simulink model "sim_5_twolink_force_control"  (R2021a)
settings: Solver=VariableStepAuto  StartTime=0.0  StopTime=15  MaxStep=1e-2
values from neighbouring files (symbols this model uses):
  b1 = 0.01    [sim_params.m]    (also in sim_params_force.m)
  b2 = 0.01    [sim_params.m]    (also in sim_params_force.m)
  D = [zeros(n); eye(n)]    [control_comparison_script.m]    (also in gen_twolink_ss.m = reshape([0.0,0.0,0.0,0.0,0.0,0.0,0.0,0.0],[4,2]))
  g = 9.80665    [sim_params.m]    (also in sim_params_force.m)
  L1x = 0.3    [sim_params.m]    (also in sim_params_force.m)
  L1y = 0.050    (= 0.05)    [sim_params.m]    (also in sim_params_force.m)
  L1z = 0.05    [sim_params.m]    (also in sim_params_force.m)
  L2x = 0.15    [sim_params.m]    (also in sim_params_force.m = 0.3)
  L2y = 0.05    [sim_params.m]    (also in sim_params_force.m)
  L2z = 0.05    [sim_params.m]    (also in sim_params_force.m)
  m1 = m1*1.25    [control_comparison_script.m]    (also in sim_params.m = 2.775; sim_params_force.m = 2.775)
  m2 = m2*1.25    [control_comparison_script.m]    (also in sim_params.m = 1.3875; sim_params_force.m = 2.775)
  max_joint_torque1 = 20    [sim_params.m]    (also in sim_params_force.m)
  max_joint_torque2 = 10    [sim_params.m]    (also in sim_params_force.m = 20)
undefined symbols (not defined in the file or in its folder): Da, KD, KD_a, Kd_p, Kd_p2, Kdt, KF, Kf_v, Kf_v2, KI, Ki_f, Ki_f2, Ki_p, Ki_p2, KP, KP_a, Kp_f, Kp_f2, Kp_p, Kp_p2, Levenberg, Ma, Marquardt, R_env, sigbuilder_block, W_env, X, Xenv, Y, Z
libraries: sm_lib x72, nesl_utility x58, pid_lib x14, simulink x3, robotmaniplib x2, robotcorelib x1
(part 1 of 6)
settings Model: Creator=Petronas-Tareq  LastModifiedBy=Petronas-Tareq
settings ExplorerConfigSet: InternalSimMechanicsExplorerSettings="<ExplorerConfiguration><canonicalview>default</canonicalview><AnimationSetting><BasePlaybackSpeed>1.0</BasePlaybackSpeed><PlaybackSpeedFactor>1.0</PlaybackSpeedFactor></AnimationSetting><TilePanel><TileInfo><Tiles Columns=\"2\" Count=\"4\" Rows=\"2\"><Column Weight=\"0.4998\"/><Column Weight=\"0.5002\"/><Row Weight=\"0.5\"/><Row Weight=\"0.5\"/><Tile Height=\"1\" Width=\"1\" X=\"0\" Y=\"0\"/><Tile Height=\"1\" Width=\"1\" X=\"0\" Y=\"1\"/><Tile Height=\"1\" Width=\"1\" X=\"1\" Y=\"0\"/><Tile Height=\"1\" Width=\"1\" X=\"1\" Y=\"1\"/></Tiles></TileInfo><SceneInfo><SceneViewer><BGColor><R>0.60000002384185791</R><G>0.60000002384185791</G><B>0.60000002384185791</B></BGColor><Camera><DoPerspective>off</DoPerspective><Position><X>0.22866161329300444</X><Y>-0.999999955971509147</Y><Z>-4.12820655437684536e-09</Z></Position><Center><X>0.22866161329300444</X><Y>4.40284908531651742e-08</Y><Z>-4.12820655437684536e-09</Z></Center><Up><X>0</X><Y>-0</Y><Z>1</Z></Up><ViewLimDist>1</ViewLimDist><YLim>0.367330397528709274</YLim><XLim>0.552253577106518345</XLim></Camera></SceneViewer><SceneViewer><BGColor><R>0.60000002384185791</R><G>0.60000002384185791</G><B>0.60000002384185791</B></BGColor><Camera><DoPerspective>off</DoPerspective><Position><X>0.204072367525804987</X><Y>-2.34335064047906805</Y><Z>0.167988192192854713</Z></Position><Center><X>0.219660802383778442</X><Y>-1.34642671678176962</Y><Z>0.0911787457755401237</Z></Center><Up><X>-0.0262288638413234881</X><Y>0.0772000539040926803</Y><Z>0.996670556592697987</Z></Up><ViewLimDist>1</ViewLimDist><YLim>0.734660795057418547</YLim><XLim>1.10450715421303669</XLim></Camera></SceneViewer><SceneViewer><BGColor><R>0.60000002384185791</R><G>0.60000002384185791</G><B>0.60000002384185791</B></BGColor><Camera><DoPerspective>off</DoPerspective><Position><X>-0.24899486320315789</X><Y>-0.765272772333560392</Y><Z>0.697835060620221048</Z></Position><Center><X>0.26973731486207464</X><Y>-0.211131790133127217</Y><Z>0.0468014982858467876</Z></Center><Up><X>0.244353234025975474</X><Y>0.633635300715601257</Y><Z>0.734028475406845016</Z></Up><ViewLimDist>1</ViewLimDist><YLim>0.614833162544433431</YLim><XLim>0.925057201179866673</XLim></Camera></SceneViewer><SceneViewer><BGColor><R>0.60000002384185791</R><G>0.60000002384185791</G><B>0.60000002384185791</B></BGColor><Camera><DoPerspective>off</DoPerspective><Position><X>0.236408339938699752</X><Y>-3.48082895840207129e-09</Y><Z>0.999999999307370047</Z></Position><Center><X>0.236408339938699752</X><Y>-3.48082895840207129e-09</Y><Z>-6.9262995339158806e-10</Z></Center><Up><X>0</X><Y>1</Y><Z>-0</Z></Up><ViewLimDist>1</ViewLimDist><YLim>0.734647572682027739</YLim><XLim>1.10532591414944359</XLim></Camera></SceneViewer></SceneInfo></TilePanel><MechEditorPanel><Cameras/><GfxPanelCameraMap/><VideoCreator><PlaybackSpeedRatio>2.0</PlaybackSpeedRatio><FrameRate>30</FrameRate><VideoFormat>Motion JPEG AVI</VideoFormat><FrameSize>auto</FrameSize></VideoCreator></MechEditorPanel></ExplorerConfiguration>"

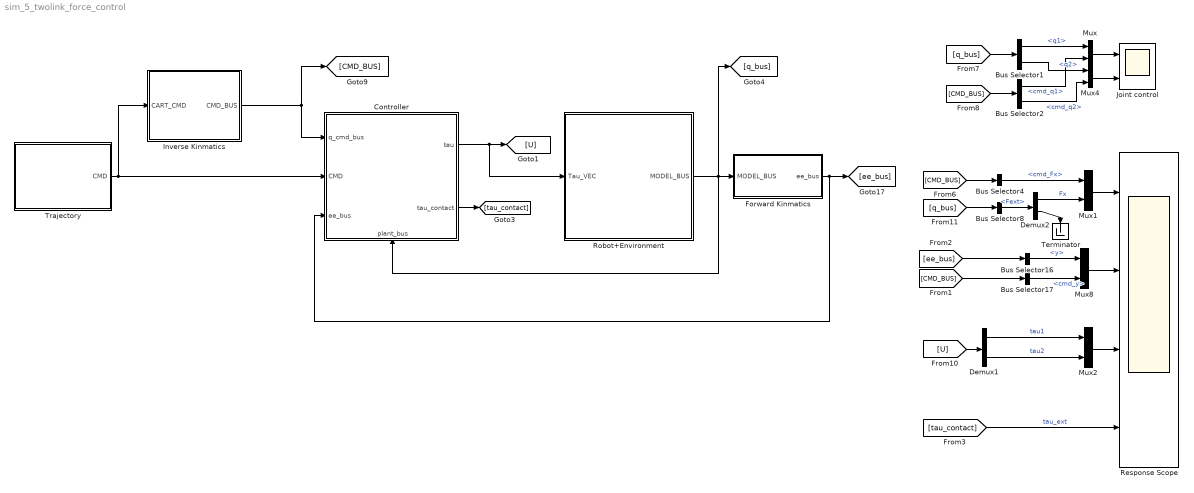
== system sim_5_twolink_force_control ==
  Bus Selector1 : BusSelector  OutputSignals=q1,q2
  Bus Selector16 : BusSelector  OutputSignals=y
  Bus Selector17 : BusSelector  OutputSignals=cmd_y
  Bus Selector2 : BusSelector  OutputSignals=cmd_q1,cmd_q2
  Bus Selector4 : BusSelector  OutputSignals=cmd_Fx
  Bus Selector8 : BusSelector  OutputSignals=Fext
  Controller : Subsystem  Variant=on  VariantControlMode=label  LabelModeActiveChoice=admittance_control  PropagateVariantConditions=on
      settings: PortSchema="{\"entries\":[{\"content\":{\"sides\":[{\"content\":{\"connectorIds\":[\"In1\",\"In2\",\"In3\"]},\"type\":\"ConnectorPlacement.EquallySpacedRectSide\",\"uuid\":\"12e0e0c2-14f8-4f2c-9d40-c223a4f2431c\"},{\"content\":{\"connectorIds\":[\"Out1\",\"Out2\"],\"side\":\"RIGHT\"},\"type\":\"ConnectorPlacement.EquallySpacedRectSide\",\"uuid\":\"b8197539-8519-4525-8d0f-ad401569c0d0\"},{\"content\":{\"connectorIds\":[],\"side\":\"TOP\"},\"type\":\"ConnectorPlacement.EquallySpacedRectSide\",\"uuid\":\"f43dc380-71af-4005-ac59-0dbedf3cc41e\"},{\"content\":{\"connectorIds\":[\"In4\"],\"side\":\"BOTTOM\"},\"type\":\"ConnectorPlacement.EquallySpacedRectSide\",\"uuid\":\"0d04f827-4285-4524-8874-ff3126ed5eeb\"}]},\"type\":\"ConnectorPlacement.EquallySpacedConnector\",\"uuid\":\"aec7d64b-efe7-424b-994a-6b7ee567ecbd\"}],\"packageUris\":[\"http://schema.mathworks.com/mf0/Connector/R2020b\"],\"version\":\"1.0\"}"
  Demux1 : Demux  Outputs=2
  Demux2 : Demux  Outputs=2
  Forward Kinmatics : Subsystem
  Inverse Kinmatics : Subsystem
  Joint control : Scope  NumInputPorts=2
  Mux{,1..2,4,8} (5 alike) : Mux  Inputs=2
  Response Scope : Scope  NumInputPorts=4
  Robot+Environment : Subsystem  Variant=on  VariantControlMode=label  LabelModeActiveChoice=Choice1
  Terminator : Terminator
  Trajectory : Subsystem  Variant=on  VariantControlMode=label  LabelModeActiveChoice=rampF-stepXY
  wires:
  Trajectory/1(CMD) -> Inverse Kinmatics/1(CART_CMD), Controller/2(CMD)
  Controller/1(tau) -> [U], Robot+Environment/1(Tau_VEC)
  Robot+Environment/1(MODEL_BUS) -> Forward Kinmatics/1(MODEL_BUS), Controller/4(plant_bus), [q_bus]
  Bus Selector2/1 -> Mux/2  "<cmd_q1>"
  Bus Selector1/2 -> Mux4/1  "<q2>"
  Mux4/1 -> Joint control/2
  [CMD_BUS] -> Bus Selector2/1
  Bus Selector1/1 -> Mux/1  "<q1>"
  Mux/1 -> Joint control/1
  Bus Selector2/2 -> Mux4/2  "<cmd_q2>"
  [q_bus] -> Bus Selector1/1
  Inverse Kinmatics/1(CMD_BUS) -> Controller/1(q_cmd_bus), [CMD_BUS]
  Bus Selector17/1 -> Mux8/2  "<cmd_y>"
  [CMD_BUS] -> Bus Selector17/1
  Bus Selector16/1 -> Mux8/1  "<y>"
  [ee_bus] -> Bus Selector16/1
  Mux8/1 -> Response Scope/2
  Forward Kinmatics/1(ee_bus) -> Controller/3(ee_bus), [ee_bus]
  Controller/2(tau_contact) -> [tau_contact]
  [tau_contact] -> Response Scope/4  "tau_ext"
  Demux1/1 -> Mux2/1  "tau1"
  [U] -> Demux1/1
  Demux1/2 -> Mux2/2  "tau2"
  Mux2/1 -> Response Scope/3
  Demux2/1 -> Mux1/2  "Fx"
  Bus Selector8/1 -> Demux2/1  "<Fext>"
  Demux2/2 -> Terminator/1
  Bus Selector4/1 -> Mux1/1  "<cmd_Fx>"
  [q_bus] -> Bus Selector8/1
  [CMD_BUS] -> Bus Selector4/1
  Mux1/1 -> Response Scope/1

== system sim_5_twolink_force_control/Controller ==
  note: 1) Add Subsystem or Model blocks as valid variant choices.
      | 2) You cannot connect blocks at this level. At simulation, connectivity is automatically
      | determined, based on the active variant and port name matching.
  q_cmd_bus : Inport
  CMD : Inport  Port=2
  ee_bus : Inport  Port=3
  plant_bus : Inport  Port=4
  Admittance+Position control : Subsystem  VariantControl=admittance_control
  "Hybrid Force/position control " : Subsystem  VariantControl=low_stiffness_hybrid
  Hybrid Force/position control (stiff) : Subsystem  VariantControl=high_stiffness_hybrid
  Parallel Force/position control (stiff) : Subsystem  VariantControl=high_stiffness_parallel
  tau : Outport
  tau_contact : Outport  Port=2

== system sim_5_twolink_force_control/Forward Kinmatics ==
  MODEL_BUS : Inport
  Bus Creator : BusCreator  Inputs=6
  Bus Selector : BusSelector  OutputSignals=q1,q2
  Bus Selector1 : BusSelector  OutputSignals=q1,q2
  Bus Selector2 : BusSelector  OutputSignals=q1_dd,q2_dd
  Bus Selector3 : BusSelector  OutputSignals=q1_d,q2_d
  Constant : Constant  Value=L1x
  Constant1 : Constant  Value=L2x
  Constant2 : Constant  Value=L1x
  Constant3 : Constant  Value=L2x
  Demux : Demux  Outputs=2
  Demux1 : Demux  Outputs=2
  Forward Kinematics : MATLAB Function  TreatAsAtomicUnit=on
  Jacobian : Subsystem
  Jacobian dot1 : Subsystem
  Jacobian1 : MATLAB Function  TreatAsAtomicUnit=on
  Matrix Multiply : Product  Multiplication=Matrix(*)
  Matrix Multiply3 : Product  Multiplication=Matrix(*)
  Matrix Multiply4 : Product  Multiplication=Matrix(*)
  Mux : Mux  Inputs=2
  Mux2 : Mux  Inputs=2
  Mux3 : Mux  Inputs=2
  Sum : Sum
  ee_bus : Outport
  wires:
  Sum/1 -> Demux1/1
  Jacobian dot1/1(J_dot) -> Matrix Multiply4/1  "J_dot"
  Constant2/1 -> Jacobian1/1(L_1)
  Bus Selector1/1 -> Mux/1, Jacobian1/3(theta_1)  "<q1>"
  Mux/1 -> Matrix Multiply/2
  Bus Selector/2 -> Forward Kinematics/4(theta_2)  "<q2>"
  Bus Selector1/2 -> Mux/2, Jacobian1/4(theta_2)  "<q2>"
  Demux/2 -> Bus Creator/2  "y_dot"
  Forward Kinematics/1(XE) -> Bus Creator/3  "x"
  Demux/1 -> Bus Creator/1  "x_dot"
  Jacobian/1(J) -> Matrix Multiply3/1
  Constant1/1 -> Forward Kinematics/2(L_2)
  Bus Creator/1 -> ee_bus/1
  Matrix Multiply/1 -> Demux/1
  Constant3/1 -> Jacobian1/2(L_2)
  Constant/1 -> Forward Kinematics/1(L_1)
  Bus Selector/1 -> Forward Kinematics/3(theta_1)  "<q1>"
  Jacobian1/1(J) -> Matrix Multiply/1  "J"
  Mux2/1 -> Matrix Multiply3/2
  Demux1/2 -> Bus Creator/6  "y_dd"
  Bus Selector3/1 -> Mux3/1  "<q1_d>"
  Bus Selector3/2 -> Mux3/2  "<q2_d>"
  Forward Kinematics/2(YE) -> Bus Creator/4  "y"
  MODEL_BUS/1 -> Bus Selector1/1, Jacobian/1(MODEL_BUS), Jacobian dot1/1(MODEL_BUS), Bus Selector3/1, Bus Selector2/1, Bus Selector/1
  Matrix Multiply3/1 -> Sum/1  "J*q_dd"
  Demux1/1 -> Bus Creator/5  "x_dd"
  Mux3/1 -> Matrix Multiply4/2
  Bus Selector2/1 -> Mux2/1  "<q1_dd>"
  Matrix Multiply4/1 -> Sum/2  "Jdot*qdot"
  Bus Selector2/2 -> Mux2/2  "<q2_dd>"

== system sim_5_twolink_force_control/Inverse Kinmatics ==
  note: Confirm IK works
  CART_CMD : Inport
  Bus Creator : BusCreator  Inputs=14
  Bus Creator1 : BusCreator  Inputs=2
  Bus Selector : BusSelector  OutputSignals=cmd_x,cmd_y
  Bus Selector1 : BusSelector  OutputSignals=cmd_x_dd,cmd_y_dd,cmd_x_d,cmd_y_d,cmd_x,cmd_y,cmd_Fx,cmd_Fy
  Bus Selector3 : BusSelector  OutputSignals=cmd_x,cmd_y
  Bus Selector4 : BusSelector  OutputSignals=x,y
  Demux : Demux  Outputs=2
  Demux1 : Demux  Outputs=2
  Demux2 : Demux  Outputs=2
  Discrete Derivative : simulink/Discrete/Discrete Derivative  gainval=1.0  ICPrevScaledInput=0.0  OutMin=[]  OutMax=[]  OutDataType=fixdt(1, 16)  OutScaling=2^-10  DoSatur=off
  Discrete Derivative1 : simulink/Discrete/Discrete Derivative  gainval=1.0  ICPrevScaledInput=0.0  OutMin=[]  OutMax=[]  OutDataType=fixdt(1, 16)  OutScaling=2^-10  DoSatur=off
  Forward Kinmatics : Subsystem
      settings: PortSchema="{\"entries\":[{\"content\":{\"sides\":[{\"content\":{\"connectorIds\":[\"In1\"]},\"type\":\"ConnectorPlacement.EquallySpacedRectSide\",\"uuid\":\"2c0f0405-b445-4922-82b0-9ed34ea6e343\"},{\"content\":{\"connectorIds\":[],\"side\":\"RIGHT\"},\"type\":\"ConnectorPlacement.EquallySpacedRectSide\",\"uuid\":\"91fea7c3-4850-470e-b524-5886f9b138cb\"},{\"content\":{\"connectorIds\":[\"Out1\"],\"side\":\"TOP\"},\"type\":\"ConnectorPlacement.EquallySpacedRectSide\",\"uuid\":\"51029b8b-093e-4a55-82a5-f93421c28d2e\"}]},\"type\":\"ConnectorPlacement.EquallySpacedConnector\",\"uuid\":\"843aee16-b8cd-4273-ac03-a5f22ed539be\"}],\"packageUris\":[\"http://schema.mathworks.com/mf0/Connector/R2020b\"],\"version\":\"1.0\"}"
  IK : Subsystem
  Mux : Mux  Inputs=2
  Scope : Scope  NumInputPorts=2
  Scope1 : Scope  NumInputPorts=6
  Scope2 : Scope  NumInputPorts=2
  CMD_BUS : Outport
  wires:
  CART_CMD/1 -> Bus Selector3/1, Bus Selector/1, Bus Selector1/1
  Bus Selector1/1 -> Bus Creator/7  "<cmd_x_dd>"
  Bus Selector1/2 -> Bus Creator/8  "<cmd_y_dd>"
  Bus Selector1/3 -> Bus Creator/9  "<cmd_x_d>"
  Bus Selector1/4 -> Bus Creator/10  "<cmd_y_d>"
  Bus Selector1/5 -> Bus Creator/11  "<cmd_x>"
  Bus Selector1/6 -> Bus Creator/12  "<cmd_y>"
  Demux1/1 -> Scope1/3, Bus Creator/3  "cmd_q1_d"
  Demux2/2 -> Scope1/6, Bus Creator/6  "cmd_q2_dd"
  Demux1/2 -> Scope1/4, Bus Creator/4  "cmd_q2_d"
  Demux/1 -> Scope1/1, Bus Creator/1  "cmd_q1"
  Demux/2 -> Scope1/2, Bus Creator/2  "cmd_q2"
  Bus Selector/1 -> IK/1(<cmd_x>)  "<cmd_x>"
  Bus Selector/2 -> IK/2(<cmd_y>)  "<cmd_y>"
  IK/1(q1) -> Bus Creator1/1, Mux/1  "q1"
  IK/2(q2) -> Bus Creator1/2, Mux/2  "q2"
  Mux/1 -> Demux/1, Discrete Derivative/1
  Discrete Derivative/1 -> Demux1/1, Discrete Derivative1/1
  Demux2/1 -> Scope1/5, Bus Creator/5  "cmd_q1_dd"
  Discrete Derivative1/1 -> Demux2/1
  Bus Creator/1 -> CMD_BUS/1
  Bus Creator1/1 -> Forward Kinmatics/1(MODEL_BUS)
  Forward Kinmatics/1(xy) -> Bus Selector4/1
  Bus Selector3/1 -> Scope/2  "<cmd_x>"
  Bus Selector4/1 -> Scope/1  "<x>"
  Bus Selector4/2 -> Scope2/1  "<y>"
  Bus Selector3/2 -> Scope2/2  "<cmd_y>"
  Bus Selector1/7 -> Bus Creator/13  "<cmd_Fx>"
  Bus Selector1/8 -> Bus Creator/14  "<cmd_Fy>"

== system sim_5_twolink_force_control/Robot+Environment ==
  note: 1) Add Subsystem or Model blocks as valid variant choices.
      | 2) You cannot connect blocks at this level. At simulation, connectivity is automatically
      | determined, based on the active variant and port name matching.
  Tau_VEC : Inport
  ARM+ Wall(complaint)  Simscape : Subsystem  VariantControl=Choice0
  ARM+Wall(stiff) Simscape : Subsystem  VariantControl=Choice1
  ARM+curve(stiff) Simscape : Subsystem  VariantControl=Choice3
  ARM+extrude(stiff) Simscape : Subsystem  VariantControl=Choice4
  ARM+no constraints Simscape : Subsystem  VariantControl=Choice5
  MODEL_BUS : Outport

== system sim_5_twolink_force_control/Trajectory ==
  note: 1) Add Subsystem or Model blocks as valid variant choices.
      | 2) You cannot connect blocks at this level. At simulation, connectivity is automatically
      | determined, based on the active variant and port name matching.
  rampFx-stepXY command : Subsystem  VariantControl=rampF-stepXY
  stepF command : Subsystem  VariantControl=stepF
  stepF-stepXY command : Subsystem  VariantControl=stepF-stepXY
  stepFx-rampY command : Subsystem  VariantControl=stepF-rampY
  CMD : Outport

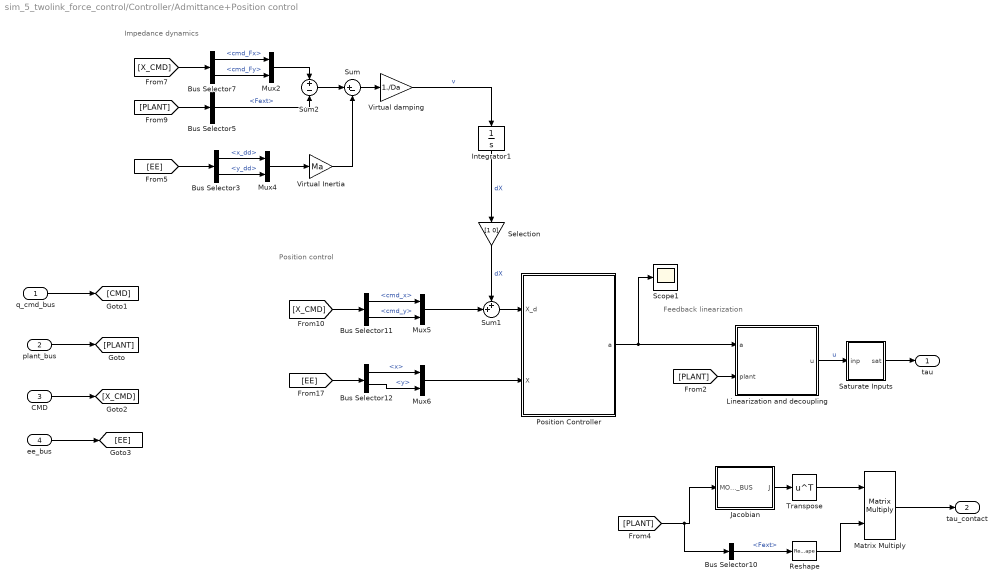
== system sim_5_twolink_force_control/Controller/Admittance+Position control ==
  note: Feedback linearization
  note: Position control
  note: Impedance dynamics
  q_cmd_bus : Inport
  plant_bus : Inport  Port=2
  CMD : Inport  Port=3
  ee_bus : Inport  Port=4
  Bus Selector10 : BusSelector  OutputSignals=Fext
  Bus Selector11 : BusSelector  OutputSignals=cmd_x,cmd_y
  Bus Selector12 : BusSelector  OutputSignals=x,y
  Bus Selector3 : BusSelector  OutputSignals=x_dd,y_dd
  Bus Selector5 : BusSelector  OutputSignals=Fext
  Bus Selector7 : BusSelector  OutputSignals=cmd_Fx,cmd_Fy
  Integrator1 : Integrator
  Jacobian : Subsystem
  Linearization and decoupling : Subsystem
  Matrix Multiply : Product  Multiplication=Matrix(*)
  Mux{2,4..6} (4 alike) : Mux  Inputs=2
  Position Controller : Subsystem
  Reshape : Reshape  OutputDimensionality=Column vector (2-D)
  Saturate Inputs : Subsystem
  Scope1 : Scope
  Selection : Gain  Gain=[1 0]
  Sum : Sum  Inputs=|+-
  Sum1 : Sum  Inputs=++|
  Sum2 : Sum  Inputs=+|-
  Transpose : Math  Operator=transpose  SaturateOnIntegerOverflow=on
  Virtual Inertia : Gain  Gain=Ma
  Virtual damping : Gain  Gain=1./Da
  tau : Outport
  tau_contact : Outport  Port=2
  wires:
  q_cmd_bus/1 -> [CMD]
  plant_bus/1 -> [PLANT]
  Transpose/1 -> Matrix Multiply/1
  CMD/1 -> [X_CMD]
  ee_bus/1 -> [EE]
  [X_CMD] -> Bus Selector11/1
  [EE] -> Bus Selector12/1
  Matrix Multiply/1 -> tau_contact/1
  Linearization and decoupling/1(u) -> Saturate Inputs/1(inp)  "u"
  Bus Selector11/1 -> Mux5/1  "<cmd_x>"
  Bus Selector11/2 -> Mux5/2  "<cmd_y>"
  Mux5/1 -> Sum1/2
  Bus Selector12/1 -> Mux6/1  "<x>"
  Bus Selector12/2 -> Mux6/2  "<y>"
  Mux6/1 -> Position Controller/2(X)
  [PLANT] -> Bus Selector10/1, Jacobian/1(MODEL_BUS)
  Bus Selector10/1 -> Reshape/1  "<Fext>"
  Jacobian/1(J) -> Transpose/1
  Reshape/1 -> Matrix Multiply/2
  Saturate Inputs/1(sat) -> tau/1
  [PLANT] -> Linearization and decoupling/2(plant)
  Virtual Inertia/1 -> Sum/2
  Bus Selector7/1 -> Mux2/1  "<cmd_Fx>"
  Bus Selector7/2 -> Mux2/2  "<cmd_Fy>"
  Sum/1 -> Virtual damping/1
  Sum2/1 -> Sum/1
  [EE] -> Bus Selector3/1
  Bus Selector3/2 -> Mux4/2  "<y_dd>"
  Bus Selector3/1 -> Mux4/1  "<x_dd>"
  Mux2/1 -> Sum2/1
  [PLANT] -> Bus Selector5/1
  Bus Selector5/1 -> Sum2/2  "<Fext>"
  [X_CMD] -> Bus Selector7/1
  Mux4/1 -> Virtual Inertia/1
  Position Controller/1(a) -> Scope1/1, Linearization and decoupling/1(a)
  Selection/1 -> Sum1/1  "dX"
  Sum1/1 -> Position Controller/1(X_d)
  Virtual damping/1 -> Integrator1/1  "v"
  Integrator1/1 -> Selection/1  "dX"

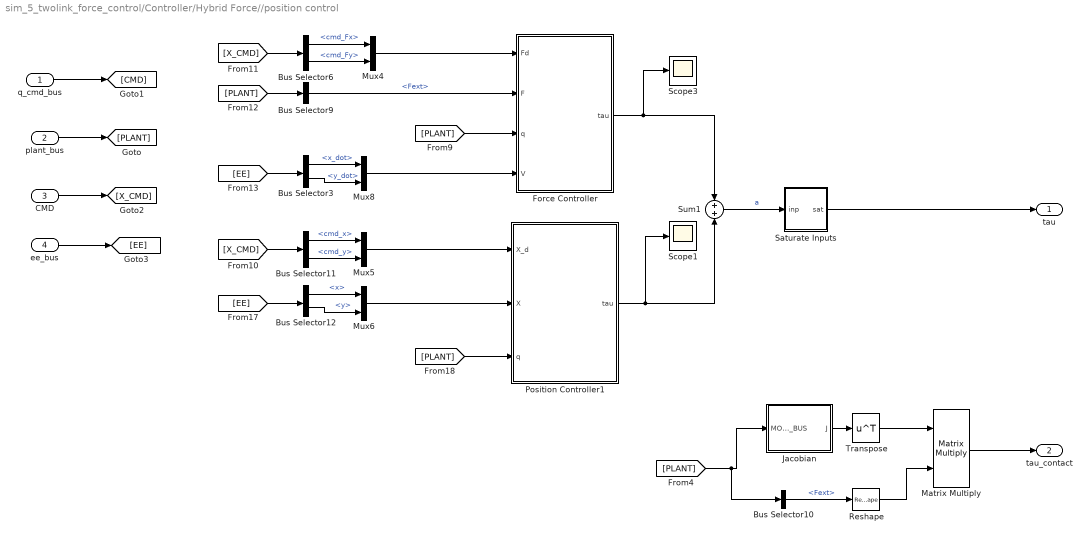
== system sim_5_twolink_force_control/Controller/Hybrid Force//position control  ==
  q_cmd_bus : Inport
  plant_bus : Inport  Port=2
  CMD : Inport  Port=3
  ee_bus : Inport  Port=4
  Bus Selector10 : BusSelector  OutputSignals=Fext
  Bus Selector11 : BusSelector  OutputSignals=cmd_x,cmd_y
  Bus Selector12 : BusSelector  OutputSignals=x,y
  Bus Selector3 : BusSelector  OutputSignals=x_dot,y_dot
  Bus Selector6 : BusSelector  OutputSignals=cmd_Fx,cmd_Fy
  Bus Selector9 : BusSelector  OutputSignals=Fext
  Force Controller : Subsystem
  Jacobian : Subsystem
  Matrix Multiply : Product  Multiplication=Matrix(*)
  Mux{4..6,8} (4 alike) : Mux  Inputs=2
  Position Controller1 : Subsystem
  Reshape : Reshape  OutputDimensionality=Column vector (2-D)
  Saturate Inputs : Subsystem
  Scope1 : Scope
  Scope3 : Scope
  Sum1 : Sum  Inputs=+|+
  Transpose : Math  Operator=transpose  SaturateOnIntegerOverflow=on
  tau : Outport
  tau_contact : Outport  Port=2
  wires:
  q_cmd_bus/1 -> [CMD]
  plant_bus/1 -> [PLANT]
  Transpose/1 -> Matrix Multiply/1
  CMD/1 -> [X_CMD]
  ee_bus/1 -> [EE]
  [X_CMD] -> Bus Selector6/1
  [PLANT] -> Bus Selector9/1
  [PLANT] -> Force Controller/3(q)
  Bus Selector9/1 -> Force Controller/2(F)  "<Fext>"
  Bus Selector6/1 -> Mux4/1  "<cmd_Fx>"
  [X_CMD] -> Bus Selector11/1
  [EE] -> Bus Selector12/1
  [PLANT] -> Position Controller1/3(q)
  Force Controller/1(tau) -> Scope3/1, Sum1/1
  Position Controller1/1(tau) -> Scope1/1, Sum1/2
  Matrix Multiply/1 -> tau_contact/1
  Sum1/1 -> Saturate Inputs/1(inp)  "a"
  Bus Selector6/2 -> Mux4/2  "<cmd_Fy>"
  Mux4/1 -> Force Controller/1(Fd)
  Bus Selector11/1 -> Mux5/1  "<cmd_x>"
  Bus Selector11/2 -> Mux5/2  "<cmd_y>"
  Mux5/1 -> Position Controller1/1(X_d)
  Bus Selector12/1 -> Mux6/1  "<x>"
  Bus Selector12/2 -> Mux6/2  "<y>"
  Mux6/1 -> Position Controller1/2(X)
  [EE] -> Bus Selector3/1
  Mux8/1 -> Force Controller/4(V)
  Bus Selector3/2 -> Mux8/2  "<y_dot>"
  Bus Selector3/1 -> Mux8/1  "<x_dot>"
  [PLANT] -> Bus Selector10/1, Jacobian/1(MODEL_BUS)
  Bus Selector10/1 -> Reshape/1  "<Fext>"
  Jacobian/1(J) -> Transpose/1
  Reshape/1 -> Matrix Multiply/2
  Saturate Inputs/1(sat) -> tau/1

== system sim_5_twolink_force_control/Controller/Hybrid Force//position control (stiff) ==
  q_cmd_bus : Inport
  plant_bus : Inport  Port=2
  CMD : Inport  Port=3
  ee_bus : Inport  Port=4
  Bus Selector10 : BusSelector  OutputSignals=Fext
  Bus Selector11 : BusSelector  OutputSignals=cmd_x,cmd_y
  Bus Selector12 : BusSelector  OutputSignals=x,y
  Bus Selector3 : BusSelector  OutputSignals=x_dot,y_dot
  Bus Selector6 : BusSelector  OutputSignals=cmd_Fx,cmd_Fy
  Bus Selector9 : BusSelector  OutputSignals=Fext
  Force Controller : Subsystem
  Jacobian : Subsystem
  Matrix Multiply : Product  Multiplication=Matrix(*)
  Mux{4..6,8} (4 alike) : Mux  Inputs=2
  Position Controller1 : Subsystem
  Reshape : Reshape  OutputDimensionality=Column vector (2-D)
  Saturate Inputs : Subsystem
  Scope1 : Scope
  Scope3 : Scope
  Sum1 : Sum  Inputs=+|+
  Transpose : Math  Operator=transpose  SaturateOnIntegerOverflow=on
  tau : Outport
  tau_contact : Outport  Port=2
  wires:
  q_cmd_bus/1 -> [CMD]
  plant_bus/1 -> [PLANT]
  Transpose/1 -> Matrix Multiply/1
  CMD/1 -> [X_CMD]
  ee_bus/1 -> [EE]
  [X_CMD] -> Bus Selector6/1
  [PLANT] -> Bus Selector9/1
  [PLANT] -> Force Controller/3(q)
  Bus Selector9/1 -> Force Controller/2(F)  "<Fext>"
  Bus Selector6/1 -> Mux4/1  "<cmd_Fx>"
  [X_CMD] -> Bus Selector11/1
  [EE] -> Bus Selector12/1
  [PLANT] -> Position Controller1/3(q)
  Force Controller/1(tau) -> Scope3/1, Sum1/1
  Position Controller1/1(tau) -> Scope1/1, Sum1/2
  Matrix Multiply/1 -> tau_contact/1
  Sum1/1 -> Saturate Inputs/1(inp)  "a"
  Bus Selector6/2 -> Mux4/2  "<cmd_Fy>"
  Mux4/1 -> Force Controller/1(Fd)
  Bus Selector11/1 -> Mux5/1  "<cmd_x>"
  Bus Selector11/2 -> Mux5/2  "<cmd_y>"
  Mux5/1 -> Position Controller1/1(X_d)
  Bus Selector12/1 -> Mux6/1  "<x>"
  Bus Selector12/2 -> Mux6/2  "<y>"
  Mux6/1 -> Position Controller1/2(X)
  [EE] -> Bus Selector3/1
  Mux8/1 -> Force Controller/4(V)
  Bus Selector3/2 -> Mux8/2  "<y_dot>"
  Bus Selector3/1 -> Mux8/1  "<x_dot>"
  [PLANT] -> Bus Selector10/1, Jacobian/1(MODEL_BUS)
  Bus Selector10/1 -> Reshape/1  "<Fext>"
  Jacobian/1(J) -> Transpose/1
  Reshape/1 -> Matrix Multiply/2
  Saturate Inputs/1(sat) -> tau/1

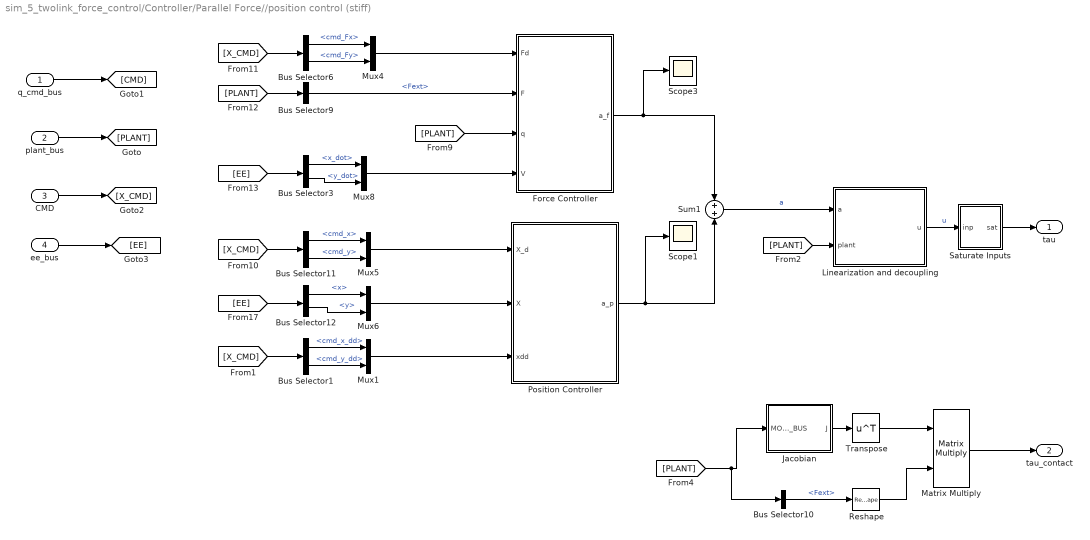
== system sim_5_twolink_force_control/Controller/Parallel Force//position control (stiff) ==
  q_cmd_bus : Inport
  plant_bus : Inport  Port=2
  CMD : Inport  Port=3
  ee_bus : Inport  Port=4
  Bus Selector1 : BusSelector  OutputSignals=cmd_x_dd,cmd_y_dd
  Bus Selector10 : BusSelector  OutputSignals=Fext
  Bus Selector11 : BusSelector  OutputSignals=cmd_x,cmd_y
  Bus Selector12 : BusSelector  OutputSignals=x,y
  Bus Selector3 : BusSelector  OutputSignals=x_dot,y_dot
  Bus Selector6 : BusSelector  OutputSignals=cmd_Fx,cmd_Fy
  Bus Selector9 : BusSelector  OutputSignals=Fext
  Force Controller : Subsystem
  Jacobian : Subsystem
  Linearization and decoupling : Subsystem
  Matrix Multiply : Product  Multiplication=Matrix(*)
  Mux{1,4..6,8} (5 alike) : Mux  Inputs=2
  Position Controller : Subsystem
  Reshape : Reshape  OutputDimensionality=Column vector (2-D)
  Saturate Inputs : Subsystem
  Scope1 : Scope
  Scope3 : Scope
  Sum1 : Sum  Inputs=+|+
  Transpose : Math  Operator=transpose  SaturateOnIntegerOverflow=on
  tau : Outport
  tau_contact : Outport  Port=2
  wires:
  q_cmd_bus/1 -> [CMD]
  plant_bus/1 -> [PLANT]
  Transpose/1 -> Matrix Multiply/1
  CMD/1 -> [X_CMD]
  ee_bus/1 -> [EE]
  [X_CMD] -> Bus Selector6/1
  [PLANT] -> Bus Selector9/1
  [PLANT] -> Force Controller/3(q)
  Bus Selector9/1 -> Force Controller/2(F)  "<Fext>"
  Bus Selector6/1 -> Mux4/1  "<cmd_Fx>"
  [X_CMD] -> Bus Selector11/1
  [EE] -> Bus Selector12/1
  Mux1/1 -> Position Controller/3(xdd)
  Force Controller/1(a_f) -> Scope3/1, Sum1/1
  Position Controller/1(a_p) -> Scope1/1, Sum1/2
  Matrix Multiply/1 -> tau_contact/1
  Linearization and decoupling/1(u) -> Saturate Inputs/1(inp)  "u"
  Bus Selector6/2 -> Mux4/2  "<cmd_Fy>"
  Mux4/1 -> Force Controller/1(Fd)
  Bus Selector11/1 -> Mux5/1  "<cmd_x>"
  Bus Selector11/2 -> Mux5/2  "<cmd_y>"
  Mux5/1 -> Position Controller/1(X_d)
  Bus Selector12/1 -> Mux6/1  "<x>"
  Bus Selector12/2 -> Mux6/2  "<y>"
  Mux6/1 -> Position Controller/2(X)
  [EE] -> Bus Selector3/1
  Mux8/1 -> Force Controller/4(V)
  Bus Selector3/2 -> Mux8/2  "<y_dot>"
  Bus Selector3/1 -> Mux8/1  "<x_dot>"
  [PLANT] -> Bus Selector10/1, Jacobian/1(MODEL_BUS)
  Bus Selector10/1 -> Reshape/1  "<Fext>"
  Jacobian/1(J) -> Transpose/1
  Reshape/1 -> Matrix Multiply/2
  Saturate Inputs/1(sat) -> tau/1
  [X_CMD] -> Bus Selector1/1
  Bus Selector1/1 -> Mux1/1  "<cmd_x_dd>"
  Bus Selector1/2 -> Mux1/2  "<cmd_y_dd>"
  Sum1/1 -> Linearization and decoupling/1(a)  "a"
  [PLANT] -> Linearization and decoupling/2(plant)

== system sim_5_twolink_force_control/Forward Kinmatics/Jacobian ==
  MODEL_BUS : Inport
  Bus Selector : BusSelector  OutputSignals=q1,q2
  Constant2 : Constant  Value=L1x
  Constant3 : Constant  Value=L2x
  Jacobian : MATLAB Function  TreatAsAtomicUnit=on
  J : Outport
  wires:
  Bus Selector/1 -> Jacobian/3(theta_1)  "<q1>"
  MODEL_BUS/1 -> Bus Selector/1
  Bus Selector/2 -> Jacobian/4(theta_2)  "<q2>"
  Constant3/1 -> Jacobian/2(L_2)
  Constant2/1 -> Jacobian/1(L_1)
  Jacobian/1(J) -> J/1  "J"

== system sim_5_twolink_force_control/Forward Kinmatics/Jacobian dot1 ==
  MODEL_BUS : Inport
  " Jacobian dot" : MATLAB Function  TreatAsAtomicUnit=on
  Bus Selector : BusSelector  OutputSignals=q1,q2,q1_d,q2_d
  Constant2 : Constant  Value=L1x
  Constant3 : Constant  Value=L2x
  J_dot : Outport
  wires:
  " Jacobian dot"/1(J_dot) -> J_dot/1  "J_dot"
  Constant2/1 -> " Jacobian dot"/1(L_1)
  Constant3/1 -> " Jacobian dot"/2(L_2)
  Bus Selector/2 -> " Jacobian dot"/4(th2)  "<q2>"
  MODEL_BUS/1 -> Bus Selector/1
  Bus Selector/1 -> " Jacobian dot"/3(th1)  "<q1>"
  Bus Selector/3 -> " Jacobian dot"/5(th1_d)  "<q1_d>"
  Bus Selector/4 -> " Jacobian dot"/6(th2_d)  "<q2_d>"

== system sim_5_twolink_force_control/Inverse Kinmatics/Forward Kinmatics ==
  MODEL_BUS : Inport
  Bus Creator : BusCreator  Inputs=2
  Bus Creator1 : BusCreator  Commented=on  Inputs=2
  Bus Selector : BusSelector  OutputSignals=q1,q2
  Constant : Constant  Value=L1x
  Constant1 : Constant  Value=L2x
  Demux3 : Demux  Commented=on  Outputs=3
  Forward Kinematics : MATLAB Function  TreatAsAtomicUnit=on
  Get Transform : robotmaniplib/Get Transform  Commented=on  RigidBodyTree=RR_robot  SourceBody=end_effector  TargetBody=base  SimulateUsing=Interpreted execution
  Mux2 : Mux  Commented=on  Inputs=2
  Reshape : Reshape  Commented=on
  Selector : Selector  Commented=on  InputPortWidth=16  IndexOptions=Index vector (dialog)  Indices=[13:15]  OutputSizes=1
  xy : Outport
  wires:
  Forward Kinematics/2(YE) -> Bus Creator/2  "y"
  Forward Kinematics/1(XE) -> Bus Creator/1  "x"
  Bus Selector/1 -> Mux2/1, Forward Kinematics/3(theta_1)  "<q1>"
  MODEL_BUS/1 -> Bus Selector/1
  Bus Selector/2 -> Mux2/2, Forward Kinematics/4(theta_2)  "<q2>"
  Constant/1 -> Forward Kinematics/1(L_1)
  Constant1/1 -> Forward Kinematics/2(L_2)
  Bus Creator/1 -> xy/1
  Mux2/1 -> Get Transform/1
  Get Transform/1 -> Reshape/1
  Reshape/1 -> Selector/1
  Selector/1 -> Demux3/1
  Demux3/1 -> Bus Creator1/1  "x"
  Demux3/2 -> Bus Creator1/2  "y"

== system sim_5_twolink_force_control/Inverse Kinmatics/IK ==
  <cmd_x> : Inport
  <cmd_y> : Inport  Port=2
  Bus Selector : BusSelector  OutputSignals=Iterations,ExitFlag
  Constant : Constant  Commented=on  Value=L1x
  Constant1 : Constant  Commented=on  Value=L2x
  Constant2 : Constant  Value=0
  Constant3 : Constant  Value=[0, 0]
  Coordinate Transformation Conversion : robotcorelib/Coordinate Transformation Conversion  InputRepresentation=Translation Vector  InputEulerSequence=ZYX  ShowTrVecInputPort=on  OutputRepresentation=Homogeneous Transformation  OutputEulerSequence=ZYX  ShowTrVecOutputPort=on  SimulateUsing=Interpreted execution
      settings: SourceProductBaseCode=RO
  Demux : Demux  Outputs=2
  IK Weights : Constant  Value=[0.1, 0.1, 0, 1, 1, 0]
  Inverse Kinematics : MATLAB Function  Commented=on  TreatAsAtomicUnit=on
  Inverse Kinematics1 : robotmaniplib/Inverse Kinematics  RigidBodyTree=RR_robot  EndEffector=end_effector  ShowInfo=on  SolverName=Levenberg-Marquardt  EnforceJointLimits=on  MaxIterations=30  MaxTime=10  GradientTolerance=1e-7  SolutionTolerance=1e-6  StepTolerance=1e-14  ErrorChangeTolerance=1e-12  UseErrorDamping=on  DampingBias=0.0025  SimulateUsing=Interpreted execution
  Mux : Mux  Inputs=3
  Scope1 : Scope
  Scope2 : Scope
  q1 : Outport
  q2 : Outport  Port=2
  wires:
  Constant1/1 -> Inverse Kinematics/4(L2)
  Constant/1 -> Inverse Kinematics/3(L1)
  <cmd_x>/1 -> Mux/1, Inverse Kinematics/1(x)
  IK Weights/1 -> Inverse Kinematics1/2
  Bus Selector/1 -> Scope2/1  "<Iterations>"
  Inverse Kinematics1/2 -> Bus Selector/1
  Coordinate Transformation Conversion/1 -> Inverse Kinematics1/1
  <cmd_y>/1 -> Inverse Kinematics/2(y), Mux/2
  Constant2/1 -> Mux/3
  Inverse Kinematics1/1 -> Demux/1
  Mux/1 -> Coordinate Transformation Conversion/1
  Bus Selector/2 -> Scope1/1  "<ExitFlag>"
  Constant3/1 -> Inverse Kinematics1/3
  Demux/2 -> q2/1  "q2_a"
  Demux/1 -> q1/1  "q1_a"

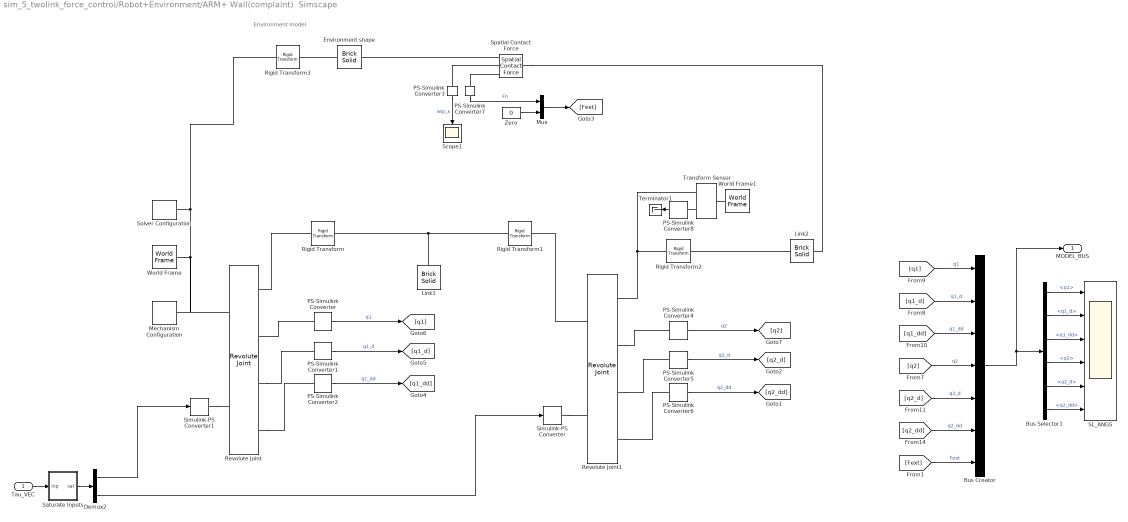
== system sim_5_twolink_force_control/Robot+Environment/ARM+ Wall(complaint)  Simscape ==
  note: Environment model
  Tau_VEC : Inport
  Bus Creator : BusCreator  Inputs=7
  Bus Selector1 : BusSelector  OutputSignals=q1,q1_d,q1_dd,q2,q2_d,q2_dd
  Demux2 : Demux  Outputs=2
  Environment shape : sm_lib/Body Elements/Brick Solid  GraphicAmbientColor=[0.15 0.15 0.15 1.0]  BasedOnType=Density  BrickDimensions=[0.04 W_env*5 0.5]  BrickDimensionUnits=m  CenterOfMass=[0 0 0]  CenterOfMassUnits=m  GraphicDiffuseColor=[1.0 0.2 0.2]  Density=density  DensityUnits=kg/m^3  DoExposeReferenceFrame=on  GraphicEmissiveColor=[0.0 0.0 0.0 1.0]  ExportEntireGeometry=on  SerializedFrames=<Frames/>  MarkerShape=Sphere  MarkerSize=10  GraphicType=FromGeometry  InertiaType=CalculateFromGeometry  Mass=1  MassUnits=kg  MomentsOfInertia=[1 1 1]  MomentsOfInertiaUnits=kg*m^2  GraphicOpacity=1.0  ProductsOfInertia=[0 0 0]  ProductsOfInertiaUnits=kg*m^2  GraphicShininess=75  GraphicSpecularColor=[0.5 0.5 0.5 1.0]  GraphicVisPropType=SimpleVisualProperties
  Link1 : sm_lib/Body Elements/Brick Solid  GraphicAmbientColor=[0.15 0.15 0.15 1.0]  BasedOnType=Density  BrickDimensions=[L1x L1y L1z]  BrickDimensionUnits=m  CenterOfMass=[0 0 0]  CenterOfMassUnits=m  GraphicDiffuseColor=[0.8 0.8 1.0]  Density=density  DensityUnits=kg/m^3  DoExposeReferenceFrame=on  GraphicEmissiveColor=[0.0 0.0 0.0 1.0]  ExportEntireGeometry=off  SerializedFrames=<Frames/>  MarkerShape=Sphere  MarkerSize=10  GraphicType=FromGeometry  InertiaType=CalculateFromGeometry  Mass=1  MassUnits=kg  MomentsOfInertia=[1 1 1]  MomentsOfInertiaUnits=kg*m^2  GraphicOpacity=1.0  ProductsOfInertia=[0 0 0]  ProductsOfInertiaUnits=kg*m^2  GraphicShininess=75  GraphicSpecularColor=[0.5 0.5 0.5 1.0]  GraphicVisPropType=SimpleVisualProperties
  Link2 : sm_lib/Body Elements/Brick Solid  GraphicAmbientColor=[0.15 0.15 0.15 1.0]  BasedOnType=Density  BrickDimensions=[L2x L2y L2z]  BrickDimensionUnits=m  CenterOfMass=[0 0 0]  CenterOfMassUnits=m  GraphicDiffuseColor=[1.0 0.6 1.0]  Density=density  DensityUnits=kg/m^3  DoExposeReferenceFrame=on  GraphicEmissiveColor=[0.0 0.0 0.0 1.0]  ExportEntireGeometry=on  SerializedFrames=<Frames/>  MarkerShape=Sphere  MarkerSize=10  GraphicType=FromGeometry  InertiaType=CalculateFromGeometry  Mass=1  MassUnits=kg  MomentsOfInertia=[1 1 1]  MomentsOfInertiaUnits=kg*m^2  GraphicOpacity=1.0  ProductsOfInertia=[0 0 0]  ProductsOfInertiaUnits=kg*m^2  GraphicShininess=75  GraphicSpecularColor=[0.5 0.5 0.5 1.0]  GraphicVisPropType=SimpleVisualProperties
  Mechanism Configuration : sm_lib/Utilities/Mechanism Configuration  UniformGravity=Constant  GravityVector=[0 -g 0 ]  GravityVectorUnits=m/s^2  GravityUnits=m/s^2  LinearizationDelta=1e-4  JointModeTransitionNonlinearIterations=2
  Mux : Mux  Inputs=2
  PS-Simulink Converter : nesl_utility/PS-Simulink Converter  PhysicalDomain=network_engine_domain  SubClassName=ps_output  LeftPortType=input  RightPortType=output  PseudoPeriodic=off  Frequencies=[]  Unit=rad  AffineConversion=off
      settings: SourceProductBaseCode=PW,SS
  PS-Simulink Converter1 : nesl_utility/PS-Simulink Converter  PhysicalDomain=network_engine_domain  SubClassName=ps_output  LeftPortType=input  RightPortType=output  PseudoPeriodic=off  Frequencies=[]  Unit=rad/s  AffineConversion=off
      settings: SourceProductBaseCode=PW,SS
  PS-Simulink Converter2 : nesl_utility/PS-Simulink Converter  PhysicalDomain=network_engine_domain  SubClassName=ps_output  LeftPortType=input  RightPortType=output  PseudoPeriodic=off  Frequencies=[]  Unit=rad/s^2  AffineConversion=off
      settings: SourceProductBaseCode=PW,SS
  PS-Simulink Converter3 : nesl_utility/PS-Simulink Converter  PhysicalDomain=network_engine_domain  SubClassName=ps_output  LeftPortType=input  RightPortType=output  PseudoPeriodic=off  Frequencies=[]  Unit=inherit  AffineConversion=off
      settings: SourceProductBaseCode=PW,SS
  PS-Simulink Converter4 : nesl_utility/PS-Simulink Converter  PhysicalDomain=network_engine_domain  SubClassName=ps_output  LeftPortType=input  RightPortType=output  PseudoPeriodic=off  Frequencies=[]  Unit=rad  AffineConversion=off
      settings: SourceProductBaseCode=PW,SS
  PS-Simulink Converter5 : nesl_utility/PS-Simulink Converter  PhysicalDomain=network_engine_domain  SubClassName=ps_output  LeftPortType=input  RightPortType=output  PseudoPeriodic=off  Frequencies=[]  Unit=rad/s  AffineConversion=off
      settings: SourceProductBaseCode=PW,SS
  PS-Simulink Converter6 : nesl_utility/PS-Simulink Converter  PhysicalDomain=network_engine_domain  SubClassName=ps_output  LeftPortType=input  RightPortType=output  PseudoPeriodic=off  Frequencies=[]  Unit=rad/s^2  AffineConversion=off
      settings: SourceProductBaseCode=PW,SS
  PS-Simulink Converter7 : nesl_utility/PS-Simulink Converter  PhysicalDomain=network_engine_domain  SubClassName=ps_output  LeftPortType=input  RightPortType=output  PseudoPeriodic=off  Frequencies=[]  Unit=inherit  AffineConversion=off
      settings: SourceProductBaseCode=PW,SS
  PS-Simulink Converter8 : nesl_utility/PS-Simulink Converter  PhysicalDomain=network_engine_domain  SubClassName=ps_output  LeftPortType=input  RightPortType=output  PseudoPeriodic=off  Frequencies=[]  Unit=1  AffineConversion=off
      settings: SourceProductBaseCode=PW,SS
  Revolute Joint : sm_lib/Joints/Revolute Joint  JointMode=Normal  SenseConstraintForce=off  SenseConstraintForceX=off  SenseConstraintForceY=off  SenseConstraintForceZ=off  SenseConstraintTorque=off  SenseConstraintTorqueX=off  SenseConstraintTorqueY=off  SenseConstraintTorqueZ=off  SenseTotalForce=off  SenseTotalForceX=off  SenseTotalForceY=off  SenseTotalForceZ=off  SenseTotalTorque=off  SenseTotalTorqueX=off  SenseTotalTorqueY=off  SenseTotalTorqueZ=off  CompositeWrenchDir=BaseOnFollower  CompositeWrenchFrame=BaseFrame  EquilibriumPosition=0  EquilibriumPositionUnits=deg  SpringStiffness=0  SpringStiffnessUnits=N*m/deg  DampingCoefficient=b1  DampingCoefficientUnits=N*m/(rad/s)  TorqueActuationMode=InputTorque  MotionActuationMode=ComputedMotion  SensePosition=on  SenseVelocity=on  SenseAcceleration=on  SenseTorqueForce=off  SenseLowerLimitTorqueForce=off  SenseUpperLimitTorqueForce=off  LowerLimitSpecify=off  LowerLimitBound=-90  LowerLimitBoundUnits=deg  LowerLimitStiffness=1e4  LowerLimitStiffnessUnits=N*m/deg  LowerLimitDamping=10  LowerLimitDampingUnits=N*m/(deg/s)  LowerLimitTransitionRegionWidth=0.1  LowerLimitTransitionRegionWidthUnits=deg  UpperLimitSpecify=off  UpperLimitBound=90  UpperLimitBoundUnits=deg  UpperLimitStiffness=1e4  UpperLimitStiffnessUnits=N*m/deg  UpperLimitDamping=10  UpperLimitDampingUnits=N*m/(deg/s)  UpperLimitTransitionRegionWidth=0.1  UpperLimitTransitionRegionWidthUnits=deg  PositionTargetSpecify=on  PositionTargetPriority=Low  PositionTargetValue=theta1_0  PositionTargetValueUnits=rad  VelocityTargetSpecify=on  VelocityTargetPriority=High  VelocityTargetValue=theta1_dot_0  VelocityTargetValueUnits=rad/s
      settings: AttributesFormatString=|
      | %<DampingCoefficient>
      | %<PositionTargetValue>
      | %<VelocityTargetValue>
  Revolute Joint1 : sm_lib/Joints/Revolute Joint  JointMode=Normal  SenseConstraintForce=off  SenseConstraintForceX=off  SenseConstraintForceY=off  SenseConstraintForceZ=off  SenseConstraintTorque=off  SenseConstraintTorqueX=off  SenseConstraintTorqueY=off  SenseConstraintTorqueZ=off  SenseTotalForce=off  SenseTotalForceX=off  SenseTotalForceY=off  SenseTotalForceZ=off  SenseTotalTorque=off  SenseTotalTorqueX=off  SenseTotalTorqueY=off  SenseTotalTorqueZ=off  CompositeWrenchDir=BaseOnFollower  CompositeWrenchFrame=FollowerFrame  EquilibriumPosition=0  EquilibriumPositionUnits=deg  SpringStiffness=0  SpringStiffnessUnits=N*m/deg  DampingCoefficient=b2  DampingCoefficientUnits=N*m/(rad/s)  TorqueActuationMode=InputTorque  MotionActuationMode=ComputedMotion  SensePosition=on  SenseVelocity=on  SenseAcceleration=on  SenseTorqueForce=off  SenseLowerLimitTorqueForce=off  SenseUpperLimitTorqueForce=off  LowerLimitSpecify=off  LowerLimitBound=-90  LowerLimitBoundUnits=deg  LowerLimitStiffness=1e4  LowerLimitStiffnessUnits=N*m/deg  LowerLimitDamping=10  LowerLimitDampingUnits=N*m/(deg/s)  LowerLimitTransitionRegionWidth=0.1  LowerLimitTransitionRegionWidthUnits=deg  UpperLimitSpecify=off  UpperLimitBound=90  UpperLimitBoundUnits=deg  UpperLimitStiffness=1e4  UpperLimitStiffnessUnits=N*m/deg  UpperLimitDamping=10  UpperLimitDampingUnits=N*m/(deg/s)  UpperLimitTransitionRegionWidth=0.1  UpperLimitTransitionRegionWidthUnits=deg  PositionTargetSpecify=on  PositionTargetPriority=Low  PositionTargetValue=theta2_0  PositionTargetValueUnits=rad  VelocityTargetSpecify=on  VelocityTargetPriority=High  VelocityTargetValue=theta2_dot_0  VelocityTargetValueUnits=rad/s
      settings: AttributesFormatString=|
      | %<DampingCoefficient>
      | %<PositionTargetValue>
      | %<VelocityTargetValue>
  Rigid Transform : sm_lib/Frames and Transforms/Rigid Transform  TranslationMethod=StandardAxis  TranslationStandardOffset=L1x/2  TranslationLengthUnit=m  TranslationStandardAxis=+X  TranslationCartesianOffset=[0 0 0]  TranslationROffset=0  TranslationROffsetUnits=m  TranslationZOffset=0  TranslationZOffsetUnits=m  TranslationThetaOffset=0  TranslationThetaOffsetUnits=deg  RotationMethod=None  RotationAngleUnits=deg  RotationStandardAxis=+Z  RotationAngle=0.0  RotationArbitraryAxis=[0 0 1]  FollAlignAxisA=+X  BaseAlignAxisA=+Y  FollAlignAxisB=+Y  BaseAlignAxisB=+Z  RotationSequenceAxes=FollowerAxes  RotationSequence=XYX  RotationSequenceAngles=[0 0 0]  RotationSequenceAnglesUnits=deg  RotationMatrix=[1 0 0; 0 1 0; 0 0 1]
  Rigid Transform1 : sm_lib/Frames and Transforms/Rigid Transform  TranslationMethod=StandardAxis  TranslationStandardOffset=L1x/2  TranslationLengthUnit=m  TranslationStandardAxis=+X  TranslationCartesianOffset=[0 0 0]  TranslationROffset=0  TranslationROffsetUnits=m  TranslationZOffset=0  TranslationZOffsetUnits=m  TranslationThetaOffset=0  TranslationThetaOffsetUnits=deg  RotationMethod=None  RotationAngleUnits=deg  RotationStandardAxis=+Z  RotationAngle=0.0  RotationArbitraryAxis=[0 0 1]  FollAlignAxisA=+X  BaseAlignAxisA=+Y  FollAlignAxisB=+Y  BaseAlignAxisB=+Z  RotationSequenceAxes=FollowerAxes  RotationSequence=XYX  RotationSequenceAngles=[0 0 0]  RotationSequenceAnglesUnits=deg  RotationMatrix=[1 0 0; 0 1 0; 0 0 1]
  Rigid Transform2 : sm_lib/Frames and Transforms/Rigid Transform  TranslationMethod=StandardAxis  TranslationStandardOffset=L2x/2  TranslationLengthUnit=m  TranslationStandardAxis=+X  TranslationCartesianOffset=[0 0 0]  TranslationROffset=0  TranslationROffsetUnits=m  TranslationZOffset=0  TranslationZOffsetUnits=m  TranslationThetaOffset=0  TranslationThetaOffsetUnits=deg  RotationMethod=None  RotationAngleUnits=deg  RotationStandardAxis=+Z  RotationAngle=0.0  RotationArbitraryAxis=[0 0 1]  FollAlignAxisA=+X  BaseAlignAxisA=+Y  FollAlignAxisB=+Y  BaseAlignAxisB=+Z  RotationSequenceAxes=FollowerAxes  RotationSequence=XYX  RotationSequenceAngles=[0 0 0]  RotationSequenceAnglesUnits=deg  RotationMatrix=[1 0 0; 0 1 0; 0 0 1]
  Rigid Transform3 : sm_lib/Frames and Transforms/Rigid Transform  TranslationMethod=StandardAxis  TranslationStandardOffset=Xenv+(L2y/2)-(1e-3)  TranslationLengthUnit=m  TranslationStandardAxis=+X  TranslationCartesianOffset=[0 0 0]  TranslationROffset=0  TranslationROffsetUnits=m  TranslationZOffset=0  TranslationZOffsetUnits=m  TranslationThetaOffset=0  TranslationThetaOffsetUnits=deg  RotationMethod=None  RotationAngleUnits=deg  RotationStandardAxis=+Z  RotationAngle=0.0  RotationArbitraryAxis=[0 0 1]  FollAlignAxisA=+X  BaseAlignAxisA=+Y  FollAlignAxisB=+Y  BaseAlignAxisB=+Z  RotationSequenceAxes=FollowerAxes  RotationSequence=XYX  RotationSequenceAngles=[0 0 0]  RotationSequenceAnglesUnits=deg  RotationMatrix=[1 0 0; 0 1 0; 0 0 1]
  SL_ANGS : Scope  NumInputPorts=6
  Saturate Inputs : Subsystem
  Scope1 : Scope
  Simulink-PS Converter : nesl_utility/Simulink-PS Converter  PhysicalDomain=network_engine_domain  SubClassName=ps_input  LeftPortType=input  RightPortType=output  PseudoPeriodic=off  Frequencies=[]  NoiseDistribution=none  NoiseParameters=[]  Unit=N*m  AffineConversion=off  FilteringAndDerivatives=zero  SimscapeFilterOrder=1  InputFilterTimeConstant=0.001  UdotUserProvided=1
      settings: SourceProductBaseCode=PW,SS
  Simulink-PS Converter1 : nesl_utility/Simulink-PS Converter  PhysicalDomain=network_engine_domain  SubClassName=ps_input  LeftPortType=input  RightPortType=output  PseudoPeriodic=off  Frequencies=[]  NoiseDistribution=none  NoiseParameters=[]  Unit=N*m  AffineConversion=off  FilteringAndDerivatives=zero  SimscapeFilterOrder=1  InputFilterTimeConstant=0.001  UdotUserProvided=1
      settings: SourceProductBaseCode=PW,SS
  Solver Configuration : nesl_utility/Solver Configuration  PhysicalDomain=network_engine_domain  SubClassName=solver  LeftPortType=input  RightPortType=generic  Tones=[]  Harmonics=[]  SimulateNoise=off  Profile=off  UseLocalSampling=off  EnableSwitchedLinearOptims=on  FrequencyDomain=off  UseCCode=off  RelTol=0.001  AbsTol=1e-06  MinStep=1e-09  ToWorkspace=off  RevertToSquareIcSolve=off  NumHomotopyIterations=100  PhasorMode=off  PhasorModeNumHarmonics=1  DoDC=off  ResidualTolerance=1e-09  UseLocalSolver=off  LocalSolverChoice=NE_TRAPEZOIDAL_ADVANCER  LocalSolverSampleTime=0.01  DoFixedCost=off  MaxNonlinIter=3  MaxModeIter=2  ComputeImpulses=off  ImpulseIterations=2  LinearAlgebra=Sparse  EquationFormulation=NE_TIME_EF  DelaysMemoryBudget=1024  AutomaticFiltering=off  FilteringTimeConstant=0.001  PartitionStorageMethod=AS_NEEDED  PartitionMemoryBudget=1024  PartitionMethod=FAST
      settings: SourceProductBaseCode=PW,SS
  Spatial Contact Force : sm_lib/Forces and Torques/Spatial Contact Force  CoefficientOfDynamicFriction=0.3  CoefficientOfStaticFriction=0.5  SenseContactBaseRotation=off  SenseContactBaseTranslation=off  NormalDamping=Ke_dc  NormalDampingUnits=N/(m/s)  SenseContactFollowerRotation=off  SenseContactFollowerTranslation=off  SenseContactSignal=off  NormalStiffness=Ke_sc  NormalStiffnessUnits=N/m  FrictionalCriticalVelocity=1e-3  FrictionalCriticalVelocityUnits=m/s  ZeroCrossDetectContactStartAndEnd=off  FrictionType=None  SenseFrictionalForceMagnitude=off  SenseNormalForceMagnitude=on  NormalForceType=SmoothSpringDamper  SenseNormalVelocity=off  SenseSeparationDistance=on  SenseTangentialVelocity=off  SenseTangentialVelocityMagnitude=off  NormalTransitionRegionWidth=1e-2  NormalTransitionRegionWidthUnits=m
  Terminator1 : Terminator
  Transform Sensor : sm_lib/Frames and Transforms/Transform Sensor  MeasurementFrame=World  SenseAngle=off  SenseAxis=off  SenseAngle1=off  SenseAngle2=off  SenseAngle3=off  SenseQ=off  SenseR=on  SenseOmegaX=off  SenseOmegaY=off  SenseOmegaZ=off  SenseOmega1=off  SenseOmega2=off  SenseOmega3=off  SenseQDot=off  SenseRDot=off  SenseAlphaX=off  SenseAlphaY=off  SenseAlphaZ=off  SenseAlpha1=off  SenseAlpha2=off  SenseAlpha3=off  SenseQDDot=off  SenseRDDot=off  SenseX=off  SenseY=off  SenseZ=off  SenseRad=off  SenseAzim=off  SenseDist=off  SenseInc=off  SenseXDot=off  SenseYDot=off  SenseZDot=off  SenseRadDot=off  SenseAzimDot=off  SenseDistDot=off  SenseIncDot=off  SenseXDDot=off  SenseYDDot=off  SenseZDDot=off  SenseRadDDot=off  SenseAzimDDot=off  SenseDistDDot=off  SenseIncDDot=off
  World Frame : sm_lib/Frames and Transforms/World Frame
  World Frame1 : sm_lib/Frames and Transforms/World Frame
  Zero : Constant  Value=0  OutDataTypeStr=Inherit: Inherit via back propagation
  MODEL_BUS : Outport
  wires:
  PS-Simulink Converter/1 -> [q1]  "q1"
  PS-Simulink Converter2/1 -> [q1_dd]  "q1_dd"
  PS-Simulink Converter1/1 -> [q1_d]  "q1_d"
  Bus Creator/1 -> Bus Selector1/1, MODEL_BUS/1
  PS-Simulink Converter4/1 -> [q2]  "q2"
  PS-Simulink Converter6/1 -> [q2_dd]  "q2_dd"
  PS-Simulink Converter5/1 -> [q2_d]  "q2_d"
  Tau_VEC/1 -> Saturate Inputs/1(inp)
  Demux2/1 -> Simulink-PS Converter1/1
  Demux2/2 -> Simulink-PS Converter/1
  Bus Selector1/2 -> SL_ANGS/2  "<q1_d>"
  Bus Selector1/5 -> SL_ANGS/5  "<q2_d>"
  Bus Selector1/6 -> SL_ANGS/6  "<q2_dd>"
  Bus Selector1/1 -> SL_ANGS/1  "<q1>"
  Bus Selector1/3 -> SL_ANGS/3  "<q1_dd>"
  [q1_dd] -> Bus Creator/3  "q1_dd"
  [q1] -> Bus Creator/1  "q1"
  [q2] -> Bus Creator/4  "q2"
  [q2_d] -> Bus Creator/5  "q2_d"
  [q1_d] -> Bus Creator/2  "q1_d"
  [q2_dd] -> Bus Creator/6  "q2_dd"
  Bus Selector1/4 -> SL_ANGS/4  "<q2>"
  PS-Simulink Converter8/1 -> Terminator1/1
  Saturate Inputs/1(sat) -> Demux2/1
  PS-Simulink Converter7/1 -> Mux/1  "Fn"
  PS-Simulink Converter3/1 -> Scope1/1  "sep_x"
  Mux/1 -> [Fext]
  Zero/1 -> Mux/2
  [Fext] -> Bus Creator/7  "Fext"
  connections:
  World Frame/RConn1 -- Revolute Joint/LConn1 -- Mechanism Configuration/RConn1 -- Rigid Transform3/LConn1 -- Solver Configuration/RConn1
  Rigid Transform1/LConn1 -- Link1/RConn1 -- Rigid Transform/RConn1
  Revolute Joint/RConn3 -- PS-Simulink Converter1/LConn1
  Revolute Joint/RConn4 -- PS-Simulink Converter2/LConn1
  Rigid Transform/LConn1 -- Revolute Joint/RConn1
  PS-Simulink Converter/LConn1 -- Revolute Joint/RConn2
  Revolute Joint1/LConn1 -- Rigid Transform1/RConn1
  Revolute Joint1/RConn3 -- PS-Simulink Converter5/LConn1
  Revolute Joint1/RConn2 -- PS-Simulink Converter4/LConn1
  Revolute Joint1/RConn4 -- PS-Simulink Converter6/LConn1
  Link2/RConn1 -- Rigid Transform2/RConn1
  Rigid Transform2/LConn1 -- Transform Sensor/RConn1 -- Revolute Joint1/RConn1
  World Frame1/RConn1 -- Transform Sensor/LConn1
  PS-Simulink Converter8/LConn1 -- Transform Sensor/RConn2
  Simulink-PS Converter/RConn1 -- Revolute Joint1/LConn2
  Simulink-PS Converter1/RConn1 -- Revolute Joint/LConn2
  Environment shape/RConn1 -- Rigid Transform3/RConn1
  Spatial Contact Force/LConn1 -- Link2/LConn1
  Spatial Contact Force/RConn1 -- Environment shape/LConn1
  PS-Simulink Converter3/LConn1 -- Spatial Contact Force/RConn2
  Spatial Contact Force/RConn3 -- PS-Simulink Converter7/LConn1
